simulink model "Drone_Control_2018b"  (R2018b)
settings: Solver=VariableStepAuto  StartTime=0.0  StopTime=100  RelTol=1e-3
libraries: simulink x3
settings Model: Creator=ewert  LastModifiedBy=21655
settings SFSimCC: SimUseLocalCustomCode=off
settings RTWCC: RTWUseLocalCustomCode=off
settings CodeAppCC: StateflowObjectComments=on

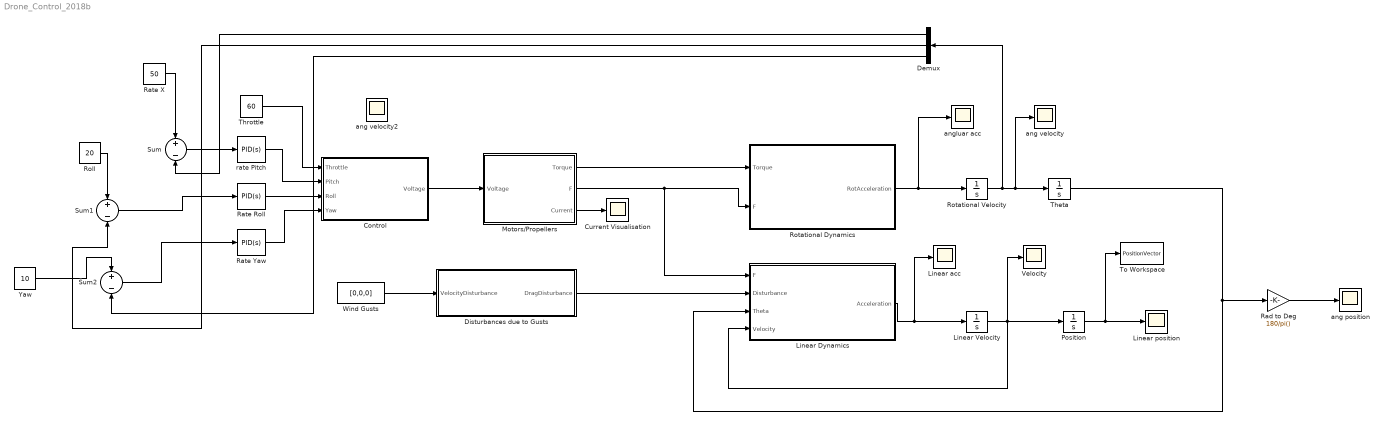
== system Drone_Control_2018b ==
  Control : MATLAB Function  TreatAsAtomicUnit=on
  "Current Visualisation " : Scope
  Demux : Demux  Outputs=3
  Disturbances due to Gusts : MATLAB Function  TreatAsAtomicUnit=on
  Linear Dynamics : MATLAB Function  TreatAsAtomicUnit=on
  Linear Velocity : Integrator
  Linear acc : Scope
  Linear position : Scope
  Motors/Propellers : MATLAB Function  TreatAsAtomicUnit=on
  Position : Integrator
  Rad to Deg : Gain  Gain=180/pi()
  Rate Roll : simulink/Continuous/PID Controller  Controller=PID  Form=Parallel  TimeDomain=Continuous-time  SampleTime=-1  IntegratorMethod=Forward Euler  ControllerParametersSource=internal  P=10  I=5  D=0  UseFilter=on  N=100  TunerSelectOption=Transfer Function Based (PID Tuner App)  InitialConditionSource=internal  InitialConditionForIntegrator=0  InitialConditionForFilter=0  DifferentiatorICPrevScaledInput=0  ExternalReset=none  TrackingMode=off  Kt=1  LimitOutput=on  UpperSaturationLimit=100  LowerSaturationLimit=0  LinearizeAsGain=on  AntiWindupMode=clamping  Kb=1  POutMin=[]  POutMax=[]  IOutMin=[]  IOutMax=[]  DOutMin=[]  DOutMax=[]  NOutMin=[]  NOutMax=[]  SumOutMin=[]  SumOutMax=[]  SaturationOutMin=[]  SaturationOutMax=[]  PParamMin=[]  PParamMax=[]  IParamMin=[]  IParamMax=[]  DParamMin=[]  DParamMax=[]  NParamMin=[]  NParamMax=[]  KbParamMin=[]  KbParamMax=[]  KtParamMin=[]  KtParamMax=[]  KbOutMin=[]  KbOutMax=[]  KtOutMin=[]  KtOutMax=[]  IntegratorOutMin=[]  IntegratorOutMax=[]  FilterOutMin=[]  FilterOutMax=[]  SumI1OutMin=[]  SumI1OutMax=[]  SumI2OutMin=[]  SumI2OutMax=[]  SumI3OutMin=[]  SumI3OutMax=[]  SumI4OutMin=[]  SumI4OutMax=[]  SumDOutMin=[]  SumDOutMax=[]  DifferentiatorOutMin=[]  DifferentiatorOutMax=[]  FilterDiffOutCoefMin=[]  FilterDiffOutCoefMax=[]  ReciprocalOutMin=[]  ReciprocalOutMax=[]  SumDenOutMin=[]  SumDenOutMax=[]  SumNumOutMin=[]  SumNumOutMax=[]  DivideOutMin=[]  DivideOutMax=[]  IntegratorContinuousStateAttributes=''  IntegratorStateMustResolveToSignalObject=off  IntegratorRTWStateStorageClass=Auto  FilterContinuousStateAttributes=''  FilterStateMustResolveToSignalObject=off  FilterRTWStateStorageClass=Auto  ParallelPVariant=InternalParameters  IdealPVariant=Disabled  IVariant=InternalParameters  DVariant=InternalParameters  IntegratorVariant=Continuous  SatVariant=Enabled  AWVariant=ContClampingParallel  PCopyVariant=Disabled  TRVariant=Disabled  FdbkBlocksVariant=Forward  IdealPFdbkVariant=Disabled  SatFdbkVariant=Disabled  DerivativeFilterVariant=ContFilter  NVariant=InternalParameters  NCopyVariant=Disabled  FilterICVariant=InternalICsFilter  IntegratorICVariant=InternalICs  ExternalResetVariant=Disabled  TRSumVariant=Passthrough  SumFdbkVariant=Disabled  SumVariant=Sum_PID
  Rate X : Constant  Value=50
  Rate Yaw : simulink/Continuous/PID Controller  Controller=PID  Form=Parallel  TimeDomain=Continuous-time  SampleTime=-1  IntegratorMethod=Forward Euler  ControllerParametersSource=internal  P=5  I=0.5  D=0  UseFilter=on  N=100  TunerSelectOption=Transfer Function Based (PID Tuner App)  InitialConditionSource=internal  InitialConditionForIntegrator=0  InitialConditionForFilter=0  DifferentiatorICPrevScaledInput=0  ExternalReset=none  TrackingMode=off  Kt=1  LimitOutput=on  UpperSaturationLimit=100  LowerSaturationLimit=0  LinearizeAsGain=on  AntiWindupMode=clamping  Kb=1  POutMin=[]  POutMax=[]  IOutMin=[]  IOutMax=[]  DOutMin=[]  DOutMax=[]  NOutMin=[]  NOutMax=[]  SumOutMin=[]  SumOutMax=[]  SaturationOutMin=[]  SaturationOutMax=[]  PParamMin=[]  PParamMax=[]  IParamMin=[]  IParamMax=[]  DParamMin=[]  DParamMax=[]  NParamMin=[]  NParamMax=[]  KbParamMin=[]  KbParamMax=[]  KtParamMin=[]  KtParamMax=[]  KbOutMin=[]  KbOutMax=[]  KtOutMin=[]  KtOutMax=[]  IntegratorOutMin=[]  IntegratorOutMax=[]  FilterOutMin=[]  FilterOutMax=[]  SumI1OutMin=[]  SumI1OutMax=[]  SumI2OutMin=[]  SumI2OutMax=[]  SumI3OutMin=[]  SumI3OutMax=[]  SumI4OutMin=[]  SumI4OutMax=[]  SumDOutMin=[]  SumDOutMax=[]  DifferentiatorOutMin=[]  DifferentiatorOutMax=[]  FilterDiffOutCoefMin=[]  FilterDiffOutCoefMax=[]  ReciprocalOutMin=[]  ReciprocalOutMax=[]  SumDenOutMin=[]  SumDenOutMax=[]  SumNumOutMin=[]  SumNumOutMax=[]  DivideOutMin=[]  DivideOutMax=[]  IntegratorContinuousStateAttributes=''  IntegratorStateMustResolveToSignalObject=off  IntegratorRTWStateStorageClass=Auto  FilterContinuousStateAttributes=''  FilterStateMustResolveToSignalObject=off  FilterRTWStateStorageClass=Auto  ParallelPVariant=InternalParameters  IdealPVariant=Disabled  IVariant=InternalParameters  DVariant=InternalParameters  IntegratorVariant=Continuous  SatVariant=Enabled  AWVariant=ContClampingParallel  PCopyVariant=Disabled  TRVariant=Disabled  FdbkBlocksVariant=Forward  IdealPFdbkVariant=Disabled  SatFdbkVariant=Disabled  DerivativeFilterVariant=ContFilter  NVariant=InternalParameters  NCopyVariant=Disabled  FilterICVariant=InternalICsFilter  IntegratorICVariant=InternalICs  ExternalResetVariant=Disabled  TRSumVariant=Passthrough  SumFdbkVariant=Disabled  SumVariant=Sum_PID
  Roll : Constant  Value=20
  Rotational Dynamics : MATLAB Function  TreatAsAtomicUnit=on
  Rotational Velocity : Integrator
  Sum : Sum  Inputs=+-
  Sum1 : Sum  Inputs=+-
  Sum2 : Sum  Inputs=+-
  Theta : Integrator
  Throttle : Constant  Value=60
  To Workspace : ToWorkspace  VariableName=PositionVector  SampleTime=-1
      settings: Save2DSignal=2-D array (concatenate along first dimension)
  "Velocity " : Scope
  Wind Gusts : Constant  Value=[0,0,0]
  Yaw : Constant  Value=10
  ang position : Scope
  ang velocity : Scope
  ang velocity2 : Scope
  angluar acc : Scope
  rate Pitch : simulink/Continuous/PID Controller  Controller=PID  Form=Parallel  TimeDomain=Continuous-time  SampleTime=-1  IntegratorMethod=Forward Euler  ControllerParametersSource=internal  P=10  I=5  D=0  UseFilter=on  N=100  TunerSelectOption=Transfer Function Based (PID Tuner App)  InitialConditionSource=internal  InitialConditionForIntegrator=0  InitialConditionForFilter=0  DifferentiatorICPrevScaledInput=0  ExternalReset=none  TrackingMode=off  Kt=1  LimitOutput=on  UpperSaturationLimit=100  LowerSaturationLimit=0  LinearizeAsGain=on  AntiWindupMode=clamping  Kb=1  POutMin=[]  POutMax=[]  IOutMin=[]  IOutMax=[]  DOutMin=[]  DOutMax=[]  NOutMin=[]  NOutMax=[]  SumOutMin=[]  SumOutMax=[]  SaturationOutMin=[]  SaturationOutMax=[]  PParamMin=[]  PParamMax=[]  IParamMin=[]  IParamMax=[]  DParamMin=[]  DParamMax=[]  NParamMin=[]  NParamMax=[]  KbParamMin=[]  KbParamMax=[]  KtParamMin=[]  KtParamMax=[]  KbOutMin=[]  KbOutMax=[]  KtOutMin=[]  KtOutMax=[]  IntegratorOutMin=[]  IntegratorOutMax=[]  FilterOutMin=[]  FilterOutMax=[]  SumI1OutMin=[]  SumI1OutMax=[]  SumI2OutMin=[]  SumI2OutMax=[]  SumI3OutMin=[]  SumI3OutMax=[]  SumI4OutMin=[]  SumI4OutMax=[]  SumDOutMin=[]  SumDOutMax=[]  DifferentiatorOutMin=[]  DifferentiatorOutMax=[]  FilterDiffOutCoefMin=[]  FilterDiffOutCoefMax=[]  ReciprocalOutMin=[]  ReciprocalOutMax=[]  SumDenOutMin=[]  SumDenOutMax=[]  SumNumOutMin=[]  SumNumOutMax=[]  DivideOutMin=[]  DivideOutMax=[]  IntegratorContinuousStateAttributes=''  IntegratorStateMustResolveToSignalObject=off  IntegratorRTWStateStorageClass=Auto  FilterContinuousStateAttributes=''  FilterStateMustResolveToSignalObject=off  FilterRTWStateStorageClass=Auto  ParallelPVariant=InternalParameters  IdealPVariant=Disabled  IVariant=InternalParameters  DVariant=InternalParameters  IntegratorVariant=Continuous  SatVariant=Enabled  AWVariant=ContClampingParallel  PCopyVariant=Disabled  TRVariant=Disabled  FdbkBlocksVariant=Forward  IdealPFdbkVariant=Disabled  SatFdbkVariant=Disabled  DerivativeFilterVariant=ContFilter  NVariant=InternalParameters  NCopyVariant=Disabled  FilterICVariant=InternalICsFilter  IntegratorICVariant=InternalICs  ExternalResetVariant=Disabled  TRSumVariant=Passthrough  SumFdbkVariant=Disabled  SumVariant=Sum_PID
  wires:
  Motors/Propellers/1(Torque) -> Rotational Dynamics/1(Torque)
  Motors/Propellers/2(F) -> Linear Dynamics/1(F), Rotational Dynamics/2(F)
  Rotational Dynamics/1(RotAcceleration) -> angluar acc/1, Rotational Velocity/1
  Rotational Velocity/1 -> Demux/1, ang velocity/1, Theta/1
  Theta/1 -> Rad to Deg/1, Linear Dynamics/3(Theta)
  Linear Dynamics/1(Acceleration) -> Linear acc/1, Linear Velocity/1
  Linear Velocity/1 -> "Velocity "/1, Position/1, Linear Dynamics/4(Velocity)
  Disturbances due to Gusts/1(DragDisturbance) -> Linear Dynamics/2(Disturbance)
  Wind Gusts/1 -> Disturbances due to Gusts/1(VelocityDisturbance)
  Control/1(Voltage) -> Motors/Propellers/1(Voltage)
  Position/1 -> To Workspace/1, Linear position/1
  Rad to Deg/1 -> ang position/1
  Motors/Propellers/3(Current) -> "Current Visualisation "/1
  Rate X/1 -> Sum/1
  Sum/1 -> rate Pitch/1
  Demux/1 -> Sum/2
  rate Pitch/1 -> Control/2(Pitch)
  Throttle/1 -> Control/1(Throttle)
  Rate Roll/1 -> Control/3(Roll)
  Roll/1 -> Sum1/1
  Sum1/1 -> Rate Roll/1
  Demux/2 -> Sum1/2
  Rate Yaw/1 -> Control/4(Yaw)
  Yaw/1 -> Sum2/1
  Sum2/1 -> Rate Yaw/1
  Demux/3 -> Sum2/2

== matlab function Drone_Control_2018b/Rotational Dynamics ==
  data: Torque input; RotAcceleration output; F input
function RotAcceleration = fcn(Torque, F)
Moment=[0 0 0];
RotAcceleration=[0 0 0];
I=[0.003,0.003,0.007];
% to keep in mind : positive torque F ( clockwise) / negative torqyue F (
% anti-clockwise)
Moment(1)=(F(3)+F(4))*0.237/2-(F(1)+F(2))*0.237/2; % moment wrt x direction (roll)
Moment(2)=(F(3)+F(2))*0.237/2-(F(1)+F(4))*0.237/2; % moment wrt y direction (putch)
Moment(3)=Torque(4)-Torque(1)+Torque(2)-Torque(3); % moment wrt z direction (yaw) 
for i=1:3
    RotAcceleration(i)=Moment(i)/I(i); % rotational acceleration = moment/moment of inertia
end

== matlab function Drone_Control_2018b/Motors//Propellers ==
  data: Voltage input; Torque output; F output; Current output
function [Torque, F, Current] = fcn(Voltage)
RPM=[0 0 0 0];
Torque=[0 0 0 0];
Current=[0 0 0 0];
F=[0 0 0 0];
for i=1:4
    RPM(i)=-2.6931*Voltage(i)^3+1400*Voltage(i);
    Ct=2*10^-15*RPM(i)^3-4*10^-11*RPM(i)^2+3*10^-7*RPM(i)+0.1013; % Thrust coefficient
    F(i)=Ct*1.225*(RPM(i)/60)^2*0.2^4; % Thrust produced by the motor/propeller couples
    Torque(i)=4*10^-14*RPM(i)^3+8*10^-12*RPM(i)^2+3*10^-6*RPM(i);
    Current(i)=1400*Torque(i); % Current pulled by motor i
end

== matlab function Drone_Control_2018b/Linear Dynamics ==
  data: F input; Acceleration output; Disturbance input; Theta input; Velocity input
function Acceleration  = fcn(F,Disturbance,Theta,Velocity)
m=0.743;
g=9.81;
A=[0.0197 0.0197 0.0512]; % projected areas
rho=1.225; % air density at sea-level 
Cd=1; % coefficient of drag

Acceleration=[0 0 0];
Force=[0 0 0];
Fprop=[0;0;0]; %thrust of propellers in the direction x, y and z

Fprop(1,1)=sin(Theta(2))*cos(Theta(1))*(F(1)+F(2)+F(3)+F(4)); % thrust in x
Fprop(2,1)=sin(Theta(1))*cos(Theta(2))*(F(1)+F(2)+F(3)+F(4)); % thrust in y

Fprop(3,1)=(F(1)+F(2)+F(3)+F(4))*cos(Theta(1))*cos(Theta(2)); % thrust in z

ThetaXY=-atan2(Fprop(1),Fprop(2));
XY2D=sqrt(Fprop(1)^2+Fprop(2)^2); % magnitude of the projection on the XY plane

% Taking Yaw motion into account
if Fprop(3)>=0 % drone pointing upwards
    Fprop(1)=XY2D*sin(Theta(3)+ThetaXY);
    Fprop(2)=XY2D*cos(Theta(3)+ThetaXY);
else
     Fprop(1)=XY2D*sin(-Theta(3)+ThetaXY);
    Fprop(2)=XY2D*cos(-Theta(3)+ThetaXY);
end
    


if Velocity(1)<0 % if the drone is moving backwards
Force(1)=Fprop(1)-Disturbance(1)+0.5*rho*Velocity(1)^2*A(1)*Cd; % add Drag
else 
    Force(1)=Fprop(1)-Disturbance(1)-0.5*rho*Velocity(1)^2*A(1)*Cd; % substract Drag
end

if Velocity(2)<0
Force(2)=Fprop(2)-Disturbance(2)+0.5*rho*Velocity(2)^2*A(2)*Cd;
else 
    Force(2)=Fprop(2)-Disturbance(2)-0.5*rho*Velocity(2)^2*A(2)*Cd;
end

if Velocity(3)<0
Force(3)=Fprop(3)+0.5*rho*Velocity(3)^2*A(3)*Cd-m*g-Disturbance(3);
else 
Force(3)=Fprop(3)-0.5*rho*Velocity(3)^2*A(3)*Cd-m*g-Disturbance(3);
end

for i=1:3 
    Acceleration(i)=Force(i)/m; % get the acceleration fron Newton's Second Law
end

== matlab function Drone_Control_2018b/Disturbances due to Gusts ==
  data: VelocityDisturbance input; DragDisturbance output
function DragDisturbance = fcn(VelocityDisturbance)
A=[0.0197 0.0197 0.0197*2*1.3];
DragDisturbance=[0 0 0];
rho=1.225;
Cd=1;

for i=1:3
    if VelocityDisturbance(i)<0
        DragDisturbance(i)=-0.5*rho*VelocityDisturbance(i)^2*A(i)*Cd;
    else
        DragDisturbance(i)=0.5*rho*VelocityDisturbance(i)^2*A(i)*Cd;
    end
end

== matlab function Drone_Control_2018b/Control ==
  data: Throttle input; Voltage output; Pitch input; Roll input; Yaw input
function Voltage = fcn(Throttle, Pitch, Roll, Yaw)
Correct=0;
if (Pitch/2+Roll/2+Yaw/2)>(100-Throttle)
    Correct=((Pitch/2+Roll/2+Yaw/2)-(100-Throttle));
end
if (Pitch/2+Roll/2+Yaw/2)>(Throttle)
    if Correct<((Pitch/2+Roll/2+Yaw/2)-(Throttle))
       Correct=((Pitch/2+Roll/2+Yaw/2)-(Throttle));
    end
end
%factors on correct to be relevant to the comparisons above which look at
%the actual application.
if Correct~=0
Pitch=Pitch-Correct/3*2;
Roll=Roll-Correct/3*2;
Yaw=Yaw-Correct/3*2;
end

Voltage=[(Throttle-Pitch/2-Roll/2-Yaw/2)*11.4/100 (Throttle-Pitch/2+Roll/2+Yaw/2)*11.4/100 (Throttle+Pitch/2+Roll/2-Yaw/2)*11.4/100 (Throttle+Pitch/2-Roll/2+Yaw/2)*11.4/100];
